simulink model "TestModell_neu"  (R2022b)
settings: Solver=FixedStepDiscrete  StartTime=0.0  StopTime=10.0  RelTol=1e-3
settings Model: Creator=lcx19  LastModifiedBy=lcx19

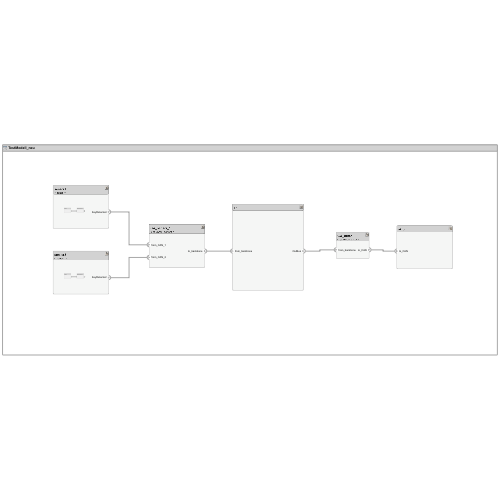
[thumbnail: Simulink's stored preview of the top-level diagram]
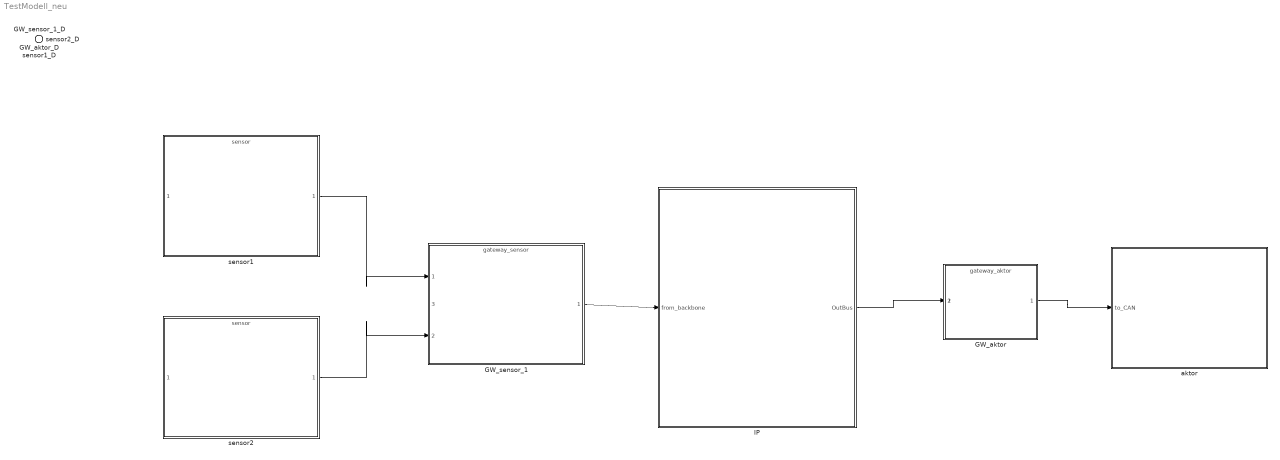
== system TestModell_neu ==
  GW_aktor_D : Inport  OutputFunctionCall=on
  GW_sensor_1_D : Inport  Port=2  OutputFunctionCall=on
  sensor1_D : Inport  Port=3  OutputFunctionCall=on
  sensor2_D : Inport  Port=4  OutputFunctionCall=on
  GW_aktor : ModelReference  ModelNameDialog=gateway_aktor  SimulationMode=Normal  ScheduleRates=on  CachedPortDiscreteRates=[-1]  ModelReferenceVersion=1.5
      settings: PortSchema="{\"entries\":[{\"content\":{\"headerSize\":38,\"margin\":15,\"minimumSpacing\":25,\"sides\":[{\"content\":{\"connectorIds\":[\"In1\"]},\"type\":\"ConnectorPlacement.EquallySpacedRectSide\",\"uuid\":\"04105025-0a3b-42e8-9b27-70a9154cf6de\"},{\"content\":{\"connectorIds\":[\"Out1\"],\"side\":\"RIGHT\"},\"type\":\"ConnectorPlacement.EquallySpacedRectSide\",\"uuid\":\"8ec2876f-44e2-4481-8f2a-65fcec53ecc3\"},{\"content\":{\"connectorIds\":[],\"side\":\"TOP\"},\"type\":\"ConnectorPlacement.EquallySpacedRectSide\",\"uuid\":\"1e3ae7a8-430e-484d-9202-f447deae3e7f\"},{\"content\":{\"connectorIds\":[\"In2\"],\"side\":\"HIDDEN\"},\"type\":\"ConnectorPlacement.EquallySpacedRectSide\",\"uuid\":\"1605ffba-ebbe-4923-aa54-068e6bbd6fab\"}]},\"type\":\"ConnectorPlacement.EquallySpacedConnector\",\"uuid\":\"b57aa59c-c581-4081-85b9-eba629c63d09\"}],\"packageUris\":[\"http://schema.mathworks.com/mf0/Connector/R2020b\"],\"version\":\"1.0\"}"
  GW_sensor_1 : ModelReference  ModelNameDialog=gateway_sensor  SimulationMode=Normal  ScheduleRates=on  CachedPortDiscreteRates=[-1]  ModelReferenceVersion=1.5
      settings: PortSchema="{\"entries\":[{\"content\":{\"headerSize\":38,\"margin\":15,\"minimumSpacing\":25,\"sides\":[{\"content\":{\"connectorIds\":[\"In1\",\"In2\"]},\"type\":\"ConnectorPlacement.EquallySpacedRectSide\",\"uuid\":\"04105025-0a3b-42e8-9b27-70a9154cf6de\"},{\"content\":{\"connectorIds\":[\"Out1\"],\"side\":\"RIGHT\"},\"type\":\"ConnectorPlacement.EquallySpacedRectSide\",\"uuid\":\"8ec2876f-44e2-4481-8f2a-65fcec53ecc3\"},{\"content\":{\"connectorIds\":[],\"side\":\"TOP\"},\"type\":\"ConnectorPlacement.EquallySpacedRectSide\",\"uuid\":\"1e3ae7a8-430e-484d-9202-f447deae3e7f\"},{\"content\":{\"connectorIds\":[\"In3\"],\"side\":\"HIDDEN\"},\"type\":\"ConnectorPlacement.EquallySpacedRectSide\",\"uuid\":\"fb395646-24dd-4536-b226-f2c57cfb1e46\"}]},\"type\":\"ConnectorPlacement.EquallySpacedConnector\",\"uuid\":\"b57aa59c-c581-4081-85b9-eba629c63d09\"}],\"packageUris\":[\"http://schema.mathworks.com/mf0/Connector/R2020b\"],\"version\":\"1.0\"}"
  IP : Subsystem
      settings: PortSchema="{\"entries\":[{\"content\":{\"headerSize\":26,\"margin\":15,\"minimumSpacing\":25,\"sides\":[{\"content\":{\"connectorIds\":[\"In1\"]},\"type\":\"ConnectorPlacement.EquallySpacedRectSide\",\"uuid\":\"c963e8d5-3700-4a3e-95ca-af085b037e50\"},{\"content\":{\"connectorIds\":[\"Out1\"],\"side\":\"RIGHT\"},\"type\":\"ConnectorPlacement.EquallySpacedRectSide\",\"uuid\":\"e55b8277-1361-4225-8557-3581b8acee68\"},{\"content\":{\"connectorIds\":[],\"side\":\"TOP\"},\"type\":\"ConnectorPlacement.EquallySpacedRectSide\",\"uuid\":\"65190ae4-2797-4c55-8402-f28e90a94a32\"}]},\"type\":\"ConnectorPlacement.EquallySpacedConnector\",\"uuid\":\"4c81c4a8-587f-43e0-b0e3-5bbe7c4f27b2\"}],\"packageUris\":[\"http://schema.mathworks.com/mf0/Connector/R2020b\"],\"version\":\"1.0\"}"
  aktor : Subsystem
      settings: PortSchema="{\"entries\":[{\"content\":{\"headerSize\":26,\"margin\":15,\"minimumSpacing\":25,\"sides\":[{\"content\":{\"connectorIds\":[\"In1\"]},\"type\":\"ConnectorPlacement.EquallySpacedRectSide\",\"uuid\":\"c963e8d5-3700-4a3e-95ca-af085b037e50\"},{\"content\":{\"connectorIds\":[],\"side\":\"RIGHT\"},\"type\":\"ConnectorPlacement.EquallySpacedRectSide\",\"uuid\":\"e55b8277-1361-4225-8557-3581b8acee68\"},{\"content\":{\"connectorIds\":[],\"side\":\"TOP\"},\"type\":\"ConnectorPlacement.EquallySpacedRectSide\",\"uuid\":\"65190ae4-2797-4c55-8402-f28e90a94a32\"}]},\"type\":\"ConnectorPlacement.EquallySpacedConnector\",\"uuid\":\"4c81c4a8-587f-43e0-b0e3-5bbe7c4f27b2\"}],\"packageUris\":[\"http://schema.mathworks.com/mf0/Connector/R2020b\"],\"version\":\"1.0\"}"
  sensor1 : ModelReference  ModelNameDialog=sensor  SimulationMode=Normal  ScheduleRates=on  CachedPortDiscreteRates=[-1]  ModelReferenceVersion=1.7
      settings: PortSchema="{\"entries\":[{\"content\":{\"headerSize\":38,\"margin\":15,\"minimumSpacing\":25,\"sides\":[{\"content\":{\"connectorIds\":[]},\"type\":\"ConnectorPlacement.EquallySpacedRectSide\",\"uuid\":\"04105025-0a3b-42e8-9b27-70a9154cf6de\"},{\"content\":{\"connectorIds\":[\"Out1\"],\"side\":\"RIGHT\"},\"type\":\"ConnectorPlacement.EquallySpacedRectSide\",\"uuid\":\"8ec2876f-44e2-4481-8f2a-65fcec53ecc3\"},{\"content\":{\"connectorIds\":[],\"side\":\"TOP\"},\"type\":\"ConnectorPlacement.EquallySpacedRectSide\",\"uuid\":\"1e3ae7a8-430e-484d-9202-f447deae3e7f\"},{\"content\":{\"connectorIds\":[\"In1\"],\"side\":\"HIDDEN\"},\"type\":\"ConnectorPlacement.EquallySpacedRectSide\",\"uuid\":\"d010d55a-c800-4a4e-817e-7dba9b93b7b4\"}]},\"type\":\"ConnectorPlacement.EquallySpacedConnector\",\"uuid\":\"b57aa59c-c581-4081-85b9-eba629c63d09\"}],\"packageUris\":[\"http://schema.mathworks.com/mf0/Connector/R2020b\"],\"version\":\"1.0\"}"
  sensor2 : ModelReference  ModelNameDialog=sensor  SimulationMode=Normal  ScheduleRates=on  CachedPortDiscreteRates=[-1]  ModelReferenceVersion=1.7
      settings: PortSchema="{\"entries\":[{\"content\":{\"headerSize\":38,\"margin\":15,\"minimumSpacing\":25,\"sides\":[{\"content\":{\"connectorIds\":[]},\"type\":\"ConnectorPlacement.EquallySpacedRectSide\",\"uuid\":\"04105025-0a3b-42e8-9b27-70a9154cf6de\"},{\"content\":{\"connectorIds\":[\"Out1\"],\"side\":\"RIGHT\"},\"type\":\"ConnectorPlacement.EquallySpacedRectSide\",\"uuid\":\"8ec2876f-44e2-4481-8f2a-65fcec53ecc3\"},{\"content\":{\"connectorIds\":[],\"side\":\"TOP\"},\"type\":\"ConnectorPlacement.EquallySpacedRectSide\",\"uuid\":\"1e3ae7a8-430e-484d-9202-f447deae3e7f\"},{\"content\":{\"connectorIds\":[\"In1\"],\"side\":\"HIDDEN\"},\"type\":\"ConnectorPlacement.EquallySpacedRectSide\",\"uuid\":\"d8315365-b274-4c56-969c-143e7c386352\"}]},\"type\":\"ConnectorPlacement.EquallySpacedConnector\",\"uuid\":\"b57aa59c-c581-4081-85b9-eba629c63d09\"}],\"packageUris\":[\"http://schema.mathworks.com/mf0/Connector/R2020b\"],\"version\":\"1.0\"}"
  wires:
  GW_sensor_1/1 -> IP/1(from_backbone)
  sensor1/1 -> GW_sensor_1/1
  sensor2/1 -> GW_sensor_1/2
  IP/1(OutBus) -> GW_aktor/1
  GW_aktor/1 -> aktor/1(to_CAN)

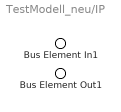
== system TestModell_neu/IP ==
  Bus Element In1 : Inport  PortName=from_backbone
  Bus Element Out1 : Outport  PortName=OutBus

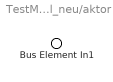
== system TestModell_neu/aktor ==
  Bus Element In1 : Inport  PortName=to_CAN
